simulink model "mpc_timevarying"  (R2023a)
settings: Solver=FixedStepDiscrete  StartTime=0.0  StopTime=5  FixedStep=Ts  RelTol=1e-3  EnableMultiTasking=on
values from neighbouring files (symbols this model uses):
  Ts = 0.1    [TimeVaryingMPCControlOfATimeVaryingLinearSystem1.m]
  x0 = zeros(size(sys.B))    [TimeVaryingMPCControlOfATimeVaryingLinearSystem1.m]
libraries: mpclib x1
settings Model: Creator=The MathWorks, Inc.  LastModifiedBy=The MathWorks, Inc.
settings SolverCC: AlgebraicLoopSolver=TrustRegion
settings DataIOCC: LimitDataPoints=on  ReturnWorkspaceOutputs=off
settings OptimizationCC: LifeSpan=inf
settings DebuggingCC: UnconnectedInputMsg=warning  UnconnectedOutputMsg=warning  UnconnectedLineMsg=warning  AllowSymbolicDim=off  SFUnexpectedBacktrackingDiag=warning  SFNoUnconditionalDefaultTransitionDiag=warning  SFExecutionAtInitializationDiag=none  ArithmeticOperatorsInVariantConditions=warning
settings ModelReferenceCC: EnableRefExpFcnMdlSchedulingChecks=on  PropagateSignalLabelsOutOfModel=off
settings SFSimCC: SimUseLocalCustomCode=off  CustomCodeUndefinedFunction=UseInterfaceOnly
settings RTWCC: RTWUseLocalCustomCode=off  DLArmComputeVersion=19.05
settings CodeAppCC: StateflowObjectComments=on
settings GRTTargetCC: TargetLangStandard=C89/C90 (ANSI)
settings ConfigComp: CovMetricSettings=dw  CovSaveCumulativeToWorkspaceVar=on  CovSaveSingleToWorkspaceVar=on  CovExternalEMLEnable=off

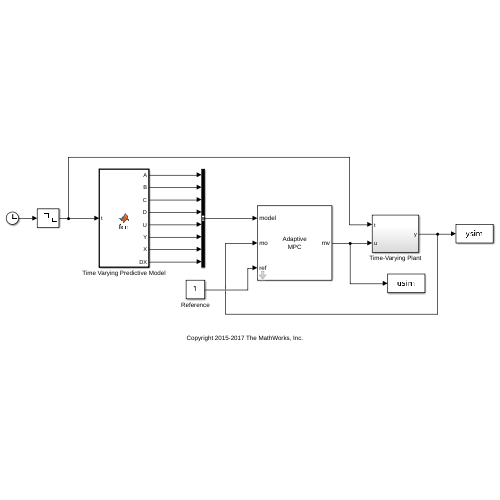
[thumbnail: Simulink's stored preview of the top-level diagram]
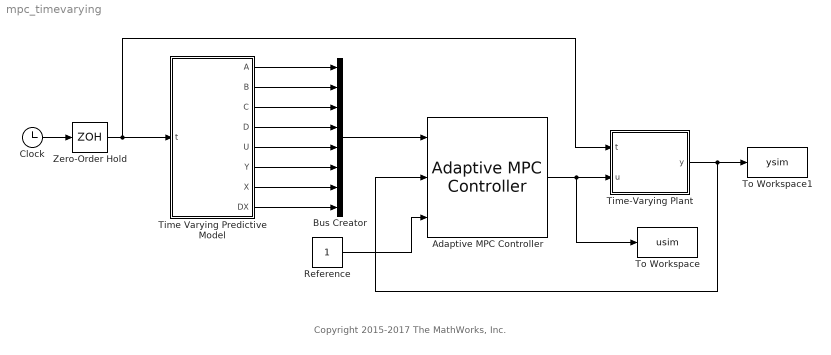
== system mpc_timevarying ==
  note: Copyright 2015-2017 The MathWorks, Inc.
  Adaptive MPC Controller : mpclib/Adaptive MPC Controller  SCDEnableBlockLinearizationSpecification=on  mpcobj=mpcobj  x0=xmpc  enable_value=0  updateMPCinCallerWorkspace=on  md_inport=off  mv_inport=off  uref_inport=off  return_cost=off  return_mvseq=off  return_qpstatus=off  return_xseq=off  return_state=off  return_ovseq=off  state_inport=off  isltv_plant=on  umin_inport=off  umax_inport=off  ymin_inport=off  ymax_inport=off  cc_inport=off  ywt_inport=off  uwt_inport=off  duwt_inport=off  rhoeps_inport=off  pm_inport=off  MaximumP=10  HorizonChoice=FixedHorizon  BlockDataType=double  SampleTimeInherited=off  switch_inport=off
  Bus Creator : BusCreator  Inputs=8
  Clock : Clock
  Reference : Constant
  Time Varying Predictive Model : MATLAB Function  TreatAsAtomicUnit=on
  Time-Varying Plant : Subsystem
  To Workspace : ToWorkspace  VariableName=usim  SampleTime=-1
  To Workspace1 : ToWorkspace  VariableName=ysim  SampleTime=-1
  Zero-Order Hold : ZeroOrderHold  SampleTime=Ts
  wires:
  Clock/1 -> Zero-Order Hold/1
  Time Varying Predictive Model/1(A) -> Bus Creator/1
  Time Varying Predictive Model/2(B) -> Bus Creator/2
  Time Varying Predictive Model/3(C) -> Bus Creator/3
  Time Varying Predictive Model/5(U) -> Bus Creator/5
  Time Varying Predictive Model/6(Y) -> Bus Creator/6
  Time Varying Predictive Model/7(X) -> Bus Creator/7
  Time Varying Predictive Model/8(DX) -> Bus Creator/8
  Time Varying Predictive Model/4(D) -> Bus Creator/4
  Bus Creator/1 -> Adaptive MPC Controller/1
  Adaptive MPC Controller/1 -> To Workspace/1, Time-Varying Plant/2(u)
  Zero-Order Hold/1 -> Time-Varying Plant/1(t), Time Varying Predictive Model/1(t)
  Time-Varying Plant/1(y) -> Adaptive MPC Controller/2, To Workspace1/1
  Reference/1 -> Adaptive MPC Controller/3

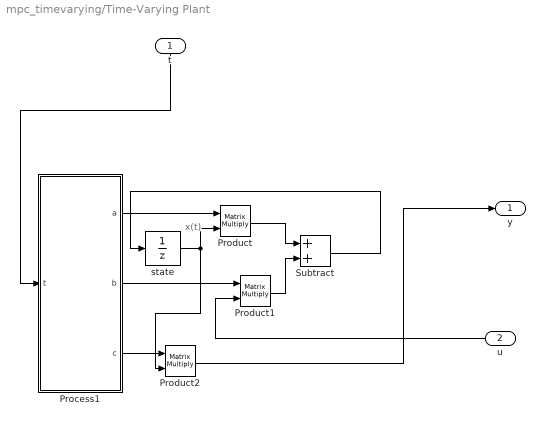
== system mpc_timevarying/Time-Varying Plant ==
  note: x(t)
  t : Inport
  u : Inport  Port=2
  Process1 : MATLAB Function  TreatAsAtomicUnit=on  SystemSampleTime=Ts
  Product : Product  Multiplication=Matrix(*)
  Product1 : Product  Multiplication=Matrix(*)
  Product2 : Product  Multiplication=Matrix(*)
  Subtract : Sum
  state : UnitDelay  InitialCondition=x0  SampleTime=Ts  HasFrameUpgradeWarning=on
  y : Outport
  wires:
  Process1/1(a) -> Product/1
  Product2/1 -> y/1
  Product/1 -> Subtract/1
  Product1/1 -> Subtract/2
  Process1/2(b) -> Product1/1
  u/1 -> Product1/2
  t/1 -> Process1/1(t)
  Process1/3(c) -> Product2/1
  state/1 -> Product/2, Product2/2
  Subtract/1 -> state/1

== matlab function mpc_timevarying/Time Varying Predictive Model ==
  data: t input; Ts parameter; A output; B output; C output; D output; U output; Y output; X output; DX output
function [A,B,C,D,U,Y,X,DX] = fcn(t,Ts)
%#codegen

coder.extrinsic('ss');
coder.extrinsic('c2d');
coder.extrinsic('tf');
coder.extrinsic('ssdata');

nx=3; % number of states
p=3;

A=zeros(nx,nx,p+1);
B=zeros(nx,1,p+1);
C=zeros(1,nx,p+1);
D=zeros(1,1,p+1);
U=zeros(1,1,p+1);
Y=zeros(1,1,p+1);
X=zeros(nx,1,p+1);
DX=zeros(nx,1,p+1);

for k=0:p,
    [a,b,c,d]=ssdata(ss(c2d(tf([5 5+2*cos((t/Ts+k)/4)],[1 3 2 6+1*sin((t/Ts+k)/2)]),Ts)));
     A(:,:,k+1)=a;
     B(:,:,k+1)=b;
     C(:,:,k+1)=c;
     D(:,:,k+1)=d;
     U(:,:,k+1)=0;
     Y(:,:,k+1)=0;
     X(:,:,k+1)=zeros(nx,1);
     DX(:,:,k+1)=zeros(nx,1);
end

== matlab function mpc_timevarying/Time-Varying Plant/Process1 ==
  data: a output; b output; t input; c output; Ts parameter
function [a,b,c] = fcn(t,Ts)
%#codegen

coder.extrinsic('ss');
coder.extrinsic('c2d');
coder.extrinsic('tf');
coder.extrinsic('ssdata');

nx=3;
a=zeros(nx,nx);
b=zeros(nx,1);
c=zeros(1,nx);

[a,b,c]=ssdata(ss(c2d(tf([5 5+2*cos(t/Ts/4)],[1 3 2 6+1*sin(t/Ts/2)]),Ts)));
